simulink model "ksp_zad16_library"  (Simulink 7.1)
settings: Solver=ode45  SolverMode=SingleTasking  StartTime=0.0  StopTime=200.0  MaxStep=0.10  RelTol=1e-3  AbsTol=1e-6
libraries: PID_continous_block x1, PID_discrete_block x1
settings Model: Creator=Slavi  LastModifiedBy=Slavi
settings SolverCC: InitialStep=0.10
settings DataIOCC: LimitDataPoints=off
settings OptimizationCC: BlockReduction=off  BooleanDataType=off
settings DebuggingCC: SaveWithParameterizedLinksMsg=none  SignalResolutionControl=TryResolveAllWithWarning  SolverPrmCheckMsg=none  MultiTaskDSMMsg=warning  MultiTaskCondExecSysMsg=none  StrictBusMsg=None
settings HardwareCC: TargetUnknown=on
settings RTWCC: IncludeERTFirstTime=on

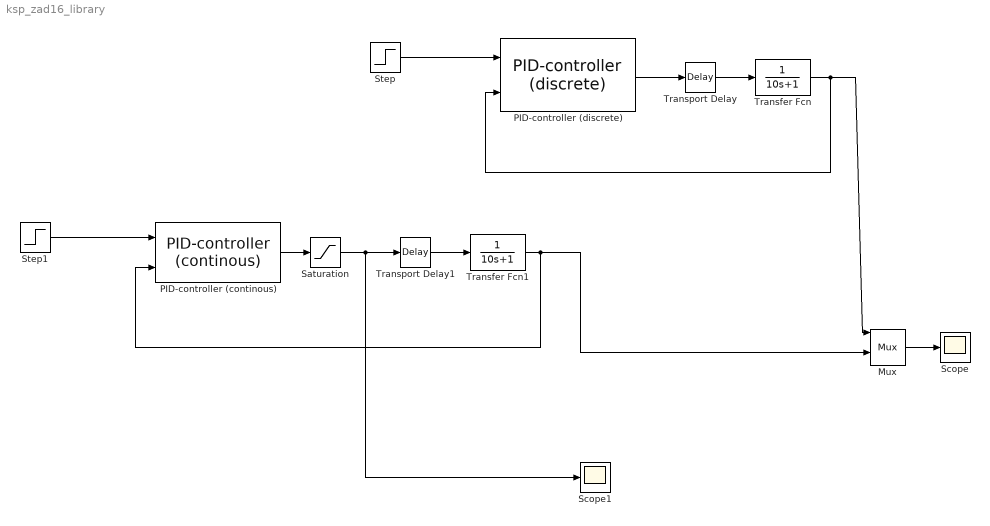
== system ksp_zad16_library ==
  Mux : Mux
  PID-controller (continous) : PID_continous_block/PID-controller (continous)  Description=PID_regulator  P=1  I=25  D=1
  PID-controller (discrete) : PID_discrete_block/PID-controller (discrete)  Description=PID_regulator  P=1  I=25  D=1  T=1
  Saturation : Saturate  UpperLimit=10  LowerLimit=-10
  Scope : Scope
      settings: TickLabels=on  YMin=-0.05  YMax=2  DataFormat=Array
  Scope1 : Scope
      settings: TickLabels=on  YMin=-10  YMax=10  DataFormat=Array
  Step : Step
  Step1 : Step
  Transfer Fcn : TransferFcn  Denominator=[10 1]
  Transfer Fcn1 : TransferFcn  Denominator=[10 1]
  Transport Delay : TransportDelay  DelayTime=2
  Transport Delay1 : TransportDelay  DelayTime=2
  wires:
  Mux/1 -> Scope/1
  Transport Delay/1 -> Transfer Fcn/1
  Step/1 -> PID-controller (discrete)/1
  Transfer Fcn/1 -> Mux/1, PID-controller (discrete)/2
  Transport Delay1/1 -> Transfer Fcn1/1
  Transfer Fcn1/1 -> PID-controller (continous)/2, Mux/3
  PID-controller (discrete)/1 -> Transport Delay/1
  Step1/1 -> PID-controller (continous)/1
  PID-controller (continous)/1 -> Saturation/1
  Saturation/1 -> Transport Delay1/1, Scope1/1
